simulink model "HW6"  (R2021a)
settings: Solver=FixedStepAuto  StartTime=0.0  StopTime=10.0  FixedStep=0.01  RelTol=1e-3
settings Model: Creator=kittithamrongaphichartkul  LastModifiedBy=thana

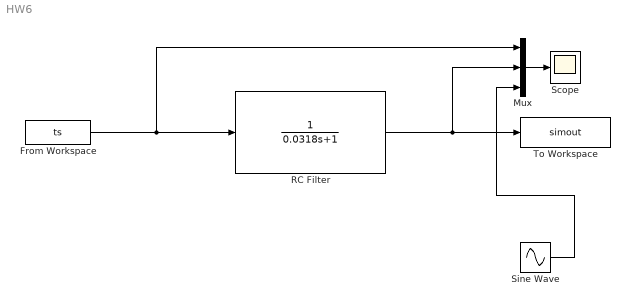
== system HW6 ==
  From Workspace : FromWorkspace  VariableName=ts
  Mux : Mux  Inputs=3
  RC Filter : TransferFcn  Denominator=[0.0318 1]
  Scope : Scope
  Sine Wave : Sin  Amplitude=1/(sqrt(2))  Frequency=2*pi*5  Phase=-pi/4  SampleTime=0
  To Workspace : ToWorkspace  VariableName=simout  SaveFormat=Timeseries  SampleTime=-1
  wires:
  From Workspace/1 -> Mux/1, RC Filter/1
  RC Filter/1 -> Mux/2, To Workspace/1
  Mux/1 -> Scope/1
  Sine Wave/1 -> Mux/3
